simulink model "vehicle_model_1"  (R2019b)
settings: Solver=VariableStepAuto  StartTime=0.0  StopTime=100  RelTol=1e-3
libraries: vrlib x3, simulink x1, mpcadaslib x1
settings Model: Creator=Owner  LastModifiedBy=Owner

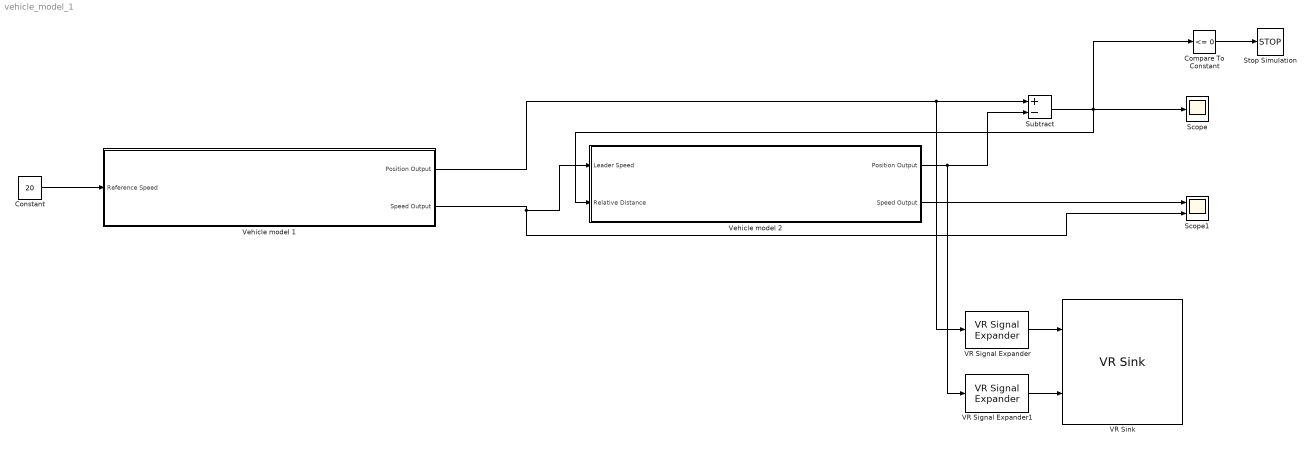
== system vehicle_model_1 ==
  Compare To Constant : simulink/Logic and Bit Operations/Compare To Constant  relop=<=  const=0  OutDataTypeStr=boolean
  Constant : Constant  Value=20
  Scope : Scope
  Scope1 : Scope  NumInputPorts=2
  Stop Simulation : Stop
  Subtract : Sum  Inputs=+-
  VR Signal Expander : vrlib/VR Signal Expander  outwidth=3  outidx=[3]
      settings: SourceProductName=Simulink
  VR Signal Expander1 : vrlib/VR Signal Expander  outwidth=3  outidx=[3]
      settings: SourceProductName=Simulink
  VR Sink : vrlib/VR Sink  InstantiateOnLoad=on  SampleTime=0.1  ViewEnable=on  RemoteChange=off  RemoteView=off  FieldsWritten=Car_Red.translation.3.1.1.double#Car_Blue.translation.3.1.1.double  WorldFileName=C:\Users\Owner\Desktop\PlatoonWorld.WRL  AutoView=off  VideoDimensions=[]  AllowVariableSize=off  FigureProperties="{'Position', 'Name', 'Viewpoint', 'CameraBound', 'CameraDirection', 'CameraPosition', 'CameraUpVector', 'ZoomFactor', 'Antialiasing', 'Headlight', 'Lighting', 'NavPanel', 'Sound', 'StatusBar', 'Stereo3D', 'Stereo3DCameraOffset', 'Stereo3DHIT', 'ToolBar', 'Textures', 'Transparency', 'Triad', 'Wireframe', 'NavZones', 'NavMode', 'NavSpeed', 'CaptureFileFormat', 'CaptureFileName', 'Record2DCompressMethod', 'Record2DCompressQuality', 'Record2D', 'Record2DFileName', 'Record2DFPS'; [7.6980000000000007e+02   8.1399999999999977e+01   7.6640000000000020e+02   6.9080000000000007e+02], '', 'Cam_CarLotus', 'on', [-2.1814319850664943e-01   0.0000000000000000e+00  -9.7591677152576595e-01], [-7.7349752524658089e-01   0.0000000000000000e+00  -1.7638817882631730e-01], [0.0000000000000000e+00   1.0000000000000000e+00   0.0000000000000000e+00], [1.0000000000000000e+00], 'on', 'on', 'on', 'halfbar', 'on', 'on', 'off', [1.0000000149011612e-01], [0.0000000000000000e+00], 'on', 'on', 'on', 'none', 'off', 'off', 'walk', 'normal', 'tif', '%f_anim_%n.tif', 'auto', [7.5000000000000000e+01], 'off', '%f_anim_%n.avi', 'auto'}"
      settings: SourceProductName=Simulink
  Vehicle model 1 : Subsystem  mask{Speed=20, Pos=100}
      mask prompts: Speed "Initial Speed"; Pos "Initial Position"
      mask TypeOptions Speed: Initial Speed/Value
      mask TypeOptions Pos: Initial Position/Value
  Vehicle model 2 : Subsystem  mask{Speed=35, Pos=0}
      mask prompts: Speed "Initial Speed"; Pos "Initial Position"
      mask TypeOptions Speed: Initial Speed/Value
      mask TypeOptions Pos: Initial Position/Value
  wires:
  Constant/1 -> Vehicle model 1/1(Reference Speed)
  Vehicle model 2/2(Speed Output) -> Scope1/1
  Vehicle model 1/2(Speed Output) -> Vehicle model 2/1(Leader Speed), Scope1/2
  Vehicle model 1/1(Position Output) -> Subtract/1, VR Signal Expander/1
  Vehicle model 2/1(Position Output) -> Subtract/2, VR Signal Expander1/1
  Subtract/1 -> Vehicle model 2/2(Relative Distance), Compare To Constant/1, Scope/1
  Compare To Constant/1 -> Stop Simulation/1
  VR Signal Expander/1 -> VR Sink/1
  VR Signal Expander1/1 -> VR Sink/2

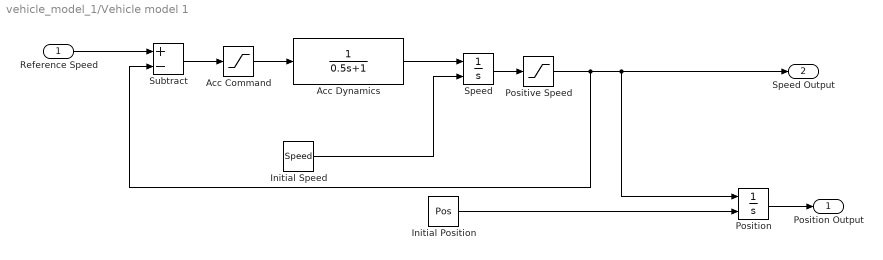
== system vehicle_model_1/Vehicle model 1 ==
  Reference Speed : Inport
  Acc Command : Saturate  UpperLimit=2  LowerLimit=-3
  Acc Dynamics : TransferFcn  Denominator=[0.5 1]
  Initial Position : Constant  Value=Pos
  Initial Speed : Constant  Value=Speed
  "Position " : Integrator  InitialConditionSource=external
  Positive Speed : Saturate  UpperLimit=inf  LowerLimit=0
  Speed : Integrator  InitialConditionSource=external
  Subtract : Sum  Inputs=+-
  Position Output : Outport
  Speed Output : Outport  Port=2
  wires:
  Subtract/1 -> Acc Command/1
  Positive Speed/1 -> Subtract/2, "Position "/1, Speed Output/1
  Acc Dynamics/1 -> Speed/1
  Reference Speed/1 -> Subtract/1
  Initial Position/1 -> "Position "/2
  Speed/1 -> Positive Speed/1
  Acc Command/1 -> Acc Dynamics/1
  Initial Speed/1 -> Speed/2
  "Position "/1 -> Position Output/1

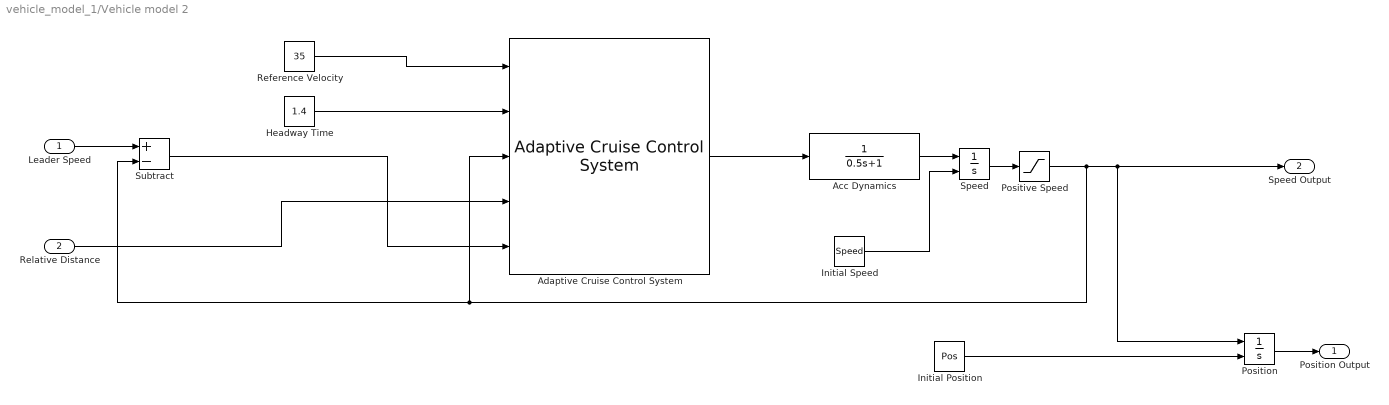
== system vehicle_model_1/Vehicle model 2 ==
  Leader Speed : Inport
  Relative Distance : Inport  Port=2
  Acc Dynamics : TransferFcn  Denominator=[0.5 1]
  Adaptive Cruise Control System : mpcadaslib/Adaptive Cruise Control System  EgoModel=tf(1,[0.5,1,0])  InitialEgoVelocity=35  DefaultSpacing=5  MaxVelocity=35  MinAcceleration=-3  amin_ext=off  MaxAcceleration=2  amax_ext=off  Ts=0.05  PredictionHorizon=200  ControllerBehavior=0.720  suboptimal=off  maxiter=10  datatypeopt=double  optmode=off  trackmode=off
      settings: SourceProductName=Model Predictive Control Toolbox
  Headway Time : Constant  Value=1.4
  Initial Position : Constant  Value=Pos
  Initial Speed : Constant  Value=Speed
  "Position " : Integrator  InitialConditionSource=external
  Positive Speed : Saturate  UpperLimit=inf  LowerLimit=0
  Reference Velocity : Constant  Value=35
  Speed : Integrator  InitialConditionSource=external
  Subtract : Sum  Inputs=+-
  Position Output : Outport
  Speed Output : Outport  Port=2
  wires:
  Positive Speed/1 -> Subtract/2, Adaptive Cruise Control System/3, "Position "/1, Speed Output/1
  Acc Dynamics/1 -> Speed/1
  Leader Speed/1 -> Subtract/1
  Initial Position/1 -> "Position "/2
  Speed/1 -> Positive Speed/1
  Initial Speed/1 -> Speed/2
  "Position "/1 -> Position Output/1
  Subtract/1 -> Adaptive Cruise Control System/5
  Relative Distance/1 -> Adaptive Cruise Control System/4
  Headway Time/1 -> Adaptive Cruise Control System/2
  Reference Velocity/1 -> Adaptive Cruise Control System/1
  Adaptive Cruise Control System/1 -> Acc Dynamics/1
